simulink model "Discrete_Controle_MISO_2019a"  (R2019a)
settings: Solver=ode3  StartTime=0.0  StopTime=12000  FixedStep=0.1  RelTol=1e-3
undefined symbols (not defined in the file or in its folder): DiscIntNeverNeededParam
libraries: simulink x2
settings Model: Creator=melol  LastModifiedBy=guima

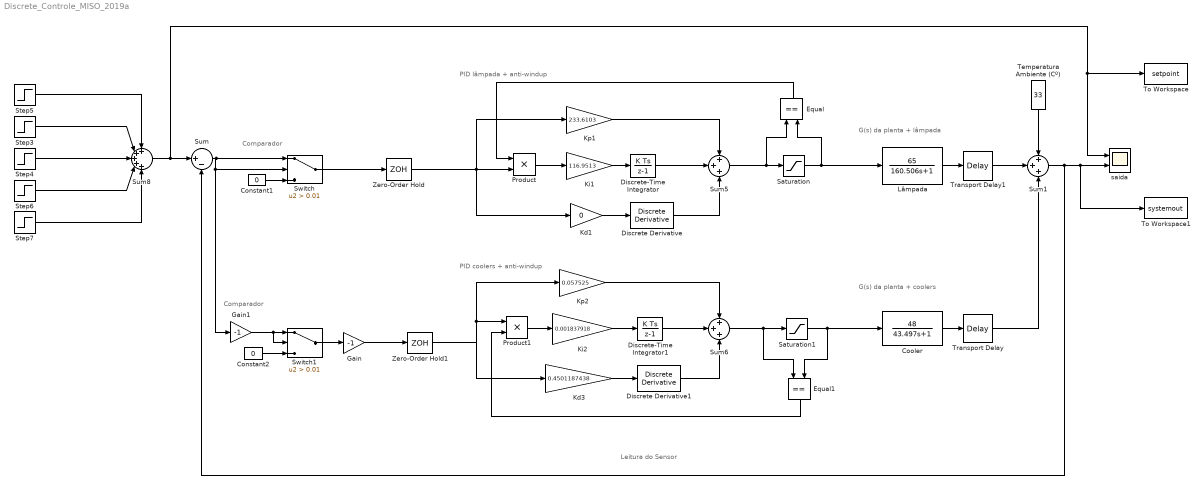
== system Discrete_Controle_MISO_2019a ==
  note: G(s) da planta + coolers
  note: G(s) da planta + lâmpada
  note: Leitura do Sensor
  note: PID coolers + anti-windup
  note: PID lâmpada + anti-windup
  note: Comparador
  note: Comparador
  Constant1 : Constant  Value=0
  Constant2 : Constant  Value=0
  Cooler : TransferFcn  Numerator=[48]  Denominator=[43.497 1]
  Discrete Derivative : simulink/Discrete/Discrete Derivative  gainval=1.0  ICPrevScaledInput=0.0  OutMin=[]  OutMax=[]  OutDataType=fixdt(1, 16)  OutScaling=2^-10  DoSatur=off
  Discrete Derivative1 : simulink/Discrete/Discrete Derivative  gainval=1.0  ICPrevScaledInput=0.0  OutMin=[]  OutMax=[]  OutDataType=fixdt(1, 16)  OutScaling=2^-10  DoSatur=off
  Discrete-Time Integrator : DiscreteIntegrator  SampleTime=-1  ICPrevOutput=DiscIntNeverNeededParam  ICPrevScaledInput=DiscIntNeverNeededParam
  Discrete-Time Integrator1 : DiscreteIntegrator  SampleTime=-1  ICPrevOutput=DiscIntNeverNeededParam  ICPrevScaledInput=DiscIntNeverNeededParam
  Equal : RelationalOperator  Operator===  OutDataTypeStr=boolean  ZeroCross=off  RndMeth=Simplest
  Equal1 : RelationalOperator  Operator===  OutDataTypeStr=boolean  ZeroCross=off  RndMeth=Simplest
  Gain : Gain  Gain=-1
  Gain1 : Gain  Gain=-1
  Kd1 : Gain  Gain=0
  Kd3 : Gain  Gain=0.4501187438
  Ki1 : Gain  Gain=116.9513
  Ki2 : Gain  Gain=0.001837918
  Kp1 : Gain  Gain=233.6103
  Kp2 : Gain  Gain=0.057525
  Lâmpada : TransferFcn  Numerator=[65]  Denominator=[160.506 1]
  Product : Product  OutDataTypeStr=double
  Product1 : Product  OutDataTypeStr=double
  Saturation : Saturate  UpperLimit=1  LowerLimit=0  ZeroCross=off
  Saturation1 : Saturate  UpperLimit=0  LowerLimit=-1  ZeroCross=off
  Step3 : Step  Time=2000  After=20  SampleTime=0
  Step4 : Step  Time=5000  After=-15  SampleTime=0
  Step5 : Step  After=35  SampleTime=0
  Step6 : Step  Time=9000  After=25  SampleTime=0
  Step7 : Step  Time=9100  After=-15  SampleTime=0
  Sum : Sum  Inputs=|+-
  Sum1 : Sum  Inputs=+++
  Sum5 : Sum  Inputs=+++
  Sum6 : Sum  Inputs=+++
  Sum8 : Sum  Inputs=+++++
  Switch : Switch  Criteria=u2 > Threshold  Threshold=0.01  ZeroCross=off
  Switch1 : Switch  Criteria=u2 > Threshold  Threshold=0.01  ZeroCross=off
  Temperatura Ambiente (Cº) : Constant  Value=33
  To Workspace : ToWorkspace  VariableName=setpoint  SaveFormat=Structure With Time  SampleTime=-1
  To Workspace1 : ToWorkspace  VariableName=systemout  SaveFormat=Structure With Time  SampleTime=-1
  Transport Delay : TransportDelay  DelayTime=17.502
  Transport Delay1 : TransportDelay  DelayTime=0
  Zero-Order Hold : ZeroOrderHold  SampleTime=-1
  Zero-Order Hold1 : ZeroOrderHold  SampleTime=-1
  "saida " : Scope  NumInputPorts=2
  wires:
  Cooler/1 -> Transport Delay/1
  Lâmpada/1 -> Transport Delay1/1
  Sum5/1 -> Equal/1, Saturation/1
  Transport Delay1/1 -> Sum1/2
  Transport Delay/1 -> Sum1/3
  Sum1/1 -> To Workspace1/1, "saida "/2, Sum/2
  Gain/1 -> Zero-Order Hold1/1
  Temperatura Ambiente (Cº)/1 -> Sum1/1
  Saturation1/1 -> Equal1/2, Cooler/1
  Saturation/1 -> Lâmpada/1, Equal/2
  Ki1/1 -> Discrete-Time Integrator/1
  Kd1/1 -> Discrete Derivative/1
  Discrete-Time Integrator/1 -> Sum5/2
  Kp1/1 -> Sum5/1
  Equal/1 -> Product/1
  Product/1 -> Ki1/1
  Kp2/1 -> Sum6/1
  Product1/1 -> Ki2/1
  Sum6/1 -> Equal1/1, Saturation1/1
  Equal1/1 -> Product1/2
  Sum8/1 -> To Workspace/1, "saida "/1, Sum/1
  Step5/1 -> Sum8/1
  Step3/1 -> Sum8/2
  Step4/1 -> Sum8/3
  Step6/1 -> Sum8/4
  Step7/1 -> Sum8/5
  Gain1/1 -> Switch1/2, Switch1/1
  Constant2/1 -> Switch1/3
  Switch1/1 -> Gain/1
  Constant1/1 -> Switch/3
  Sum/1 -> Gain1/1, Switch/2, Switch/1
  Zero-Order Hold/1 -> Kd1/1, Kp1/1, Product/2
  Switch/1 -> Zero-Order Hold/1
  Zero-Order Hold1/1 -> Kp2/1, Kd3/1, Product1/1
  Discrete Derivative/1 -> Sum5/3
  Ki2/1 -> Discrete-Time Integrator1/1
  Kd3/1 -> Discrete Derivative1/1
  Discrete-Time Integrator1/1 -> Sum6/2
  Discrete Derivative1/1 -> Sum6/3
